simulink model "CL_NL_DH_18_jun_2026"  (R2025b)
settings: Solver=ode4  StartTime=0.0  StopTime=150  FixedStep=Ts  RelTol=1e-3
values from neighbouring files (symbols this model uses):
  att_alt = 0    [guiagem_NL.m]
  coef_Ana = 1    [guiagem_NL.m]
  coef_Sato = 0    [guiagem_NL.m]
  i = find([Plantas.Ve] == VT_missao & [Plantas.He] == 600, 1)    [guiagem_NL.m]
  phi_psi = 0    [guiagem_NL.m]
  surfaces = 24    [guiagem_NL.m]
  Variacao_Iner = 0    [guiagem_NL.m]
  VT_Throttle = 1    [guiagem_NL.m]
undefined symbols (not defined in the file or in its folder): Plantas, refAlt, refPhi, refPsi, reftheta
libraries: simulink_extras x14
settings Model: SimulationMode=accelerator  Creator=mirko  LastModifiedBy=mirko

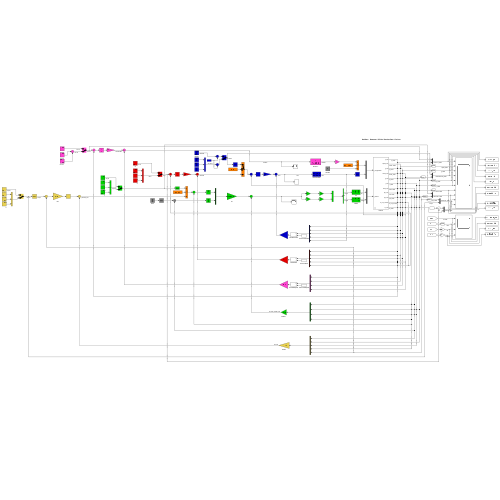
[thumbnail: Simulink's stored preview of the top-level diagram]
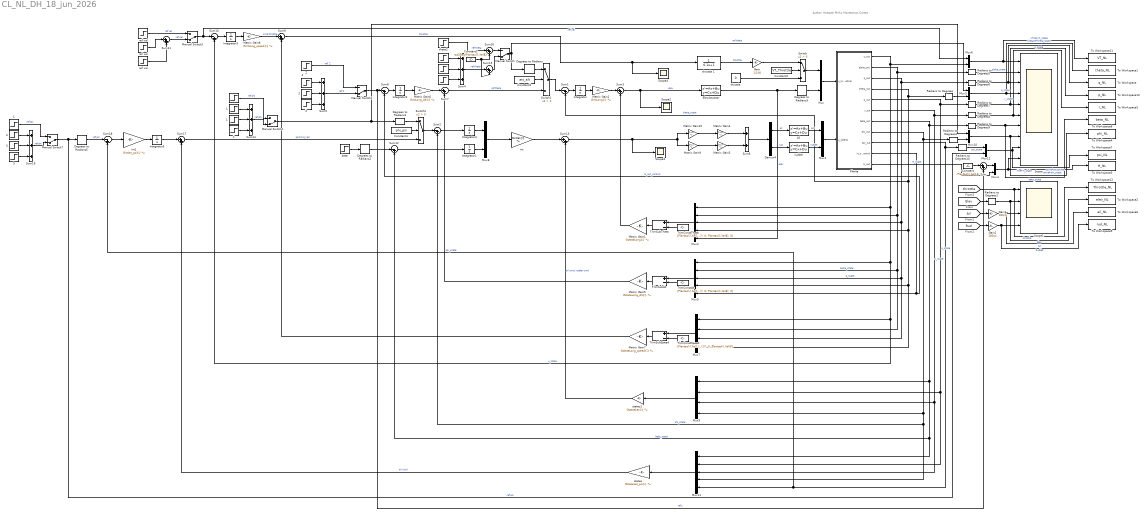
== system CL_NL_DH_18_jun_2026 ==
  note: Author: Huascar Mirko Montecinos Cortez
  "   " : Step  Time=80  After=refPhi  SampleTime=0
  "     " : Step  Time=40  After=reftheta  SampleTime=0
  "          " : Step  Time=80  Before=-reftheta  After=0  SampleTime=0
  "            " : Step  Time=60  Before=reftheta  After=-reftheta  SampleTime=0
  "            1" : Step  Time=110  Before=refPhi  After=-refPhi  SampleTime=0
  "            2" : Step  Time=60  Before=refAlt  After=-refAlt  SampleTime=0
  "            3" : Step  Time=110  Before=refPsi  After=-refPsi  SampleTime=0
  "          1" : Step  Time=130  Before=-refPhi  After=0  SampleTime=0
  "          2" : Step  Time=80  Before=-refAlt  After=0  SampleTime=0
  "          3" : Step  Time=130  Before=-refPsi  After=0  SampleTime=0
  "     1" : Step  Time=90  After=refPhi  SampleTime=0
  "     2" : Step  Time=40  After=refAlt  SampleTime=0
  "     3" : Step  Time=90  After=refPsi  SampleTime=0
  "   1" : Step  Time=80  After=refPsi  SampleTime=0
  " Z " : Step  Time=40  After=refAlt  SampleTime=0
  " ref vel " : Step  Time=5  Before=Plantas(i).Xe(1)  After=Plantas(i).Xe(1)  SampleTime=0
  Ail : StateSpace  A=-surfaces  B=surfaces  D=0  InitialCondition=0
  Constant : Constant  Value=-Plantas(i).Xe(12)
  Constant1 : Constant  Value=rad2deg(Plantas(i).Xe(8))
  Constant2 : Constant  Value=VT_Throttle
  Constant3 : Constant  Value=att_alt
  Constant4 : Constant  Value=phi_psi
  Degrees to Radians{,1..3,5} (5 alike) : simulink_extras/Transformations/Degrees to Radians
  Demux4 : Demux  Outputs=2
      settings: DisplayOption=none
  ElevActuator : StateSpace  A=-surfaces  B=surfaces  D=0  InitialCondition=Plantas(i).Ue(2)
  Gain : Gain  Gain=1/100
  Gain1 : Gain  Gain=180/pi
  Gain2 : Gain  Gain=180/pi
  Integrator{,1..5} (6 alike) : Integrator
  Manual Switch{,2..4,7} (5 alike) : ManualSwitch  CurrentSetting=0
  Matrix Gain1 : Gain  Gain=GstateLong{i}  Multiplication=Matrix(K*u)  SaturateOnIntegerOverflow=on  OutDataTypeStr=Inherit: Same as input  ParamDataTypeStr=Inherit: Same as input
  Matrix Gain10 : Gain  Gain=[1 0]  Multiplication=Matrix(K*u)  SaturateOnIntegerOverflow=on  OutDataTypeStr=Inherit: Same as input  ParamDataTypeStr=Inherit: Same as input
  Matrix Gain2 : Gain  Gain=GintLong{i}  Multiplication=Matrix(K*u)  SaturateOnIntegerOverflow=on  OutDataTypeStr=Inherit: Same as input  ParamDataTypeStr=Inherit: Same as input
  Matrix Gain3 : Gain  Gain=[0 1]'  Multiplication=Matrix(K*u)  SaturateOnIntegerOverflow=on  OutDataTypeStr=Inherit: Same as input  ParamDataTypeStr=Inherit: Same as input
  Matrix Gain4 : Gain  Gain=[1 0]'  Multiplication=Matrix(K*u)  SaturateOnIntegerOverflow=on  OutDataTypeStr=Inherit: Same as input  ParamDataTypeStr=Inherit: Same as input
  Matrix Gain5 : Gain  Gain=GstateLong_Alt{i}  Multiplication=Matrix(K*u)  SaturateOnIntegerOverflow=on  OutDataTypeStr=Inherit: Same as input  ParamDataTypeStr=Inherit: Same as input
  Matrix Gain6 : Gain  Gain=GintLong_Alt{i}  Multiplication=Matrix(K*u)  SaturateOnIntegerOverflow=on  OutDataTypeStr=Inherit: Same as input  ParamDataTypeStr=Inherit: Same as input
  Matrix Gain7 : Gain  Gain=GstateLong_speed{i}  Multiplication=Matrix(K*u)  SaturateOnIntegerOverflow=on  OutDataTypeStr=Inherit: Same as input  ParamDataTypeStr=Inherit: Same as input
  Matrix Gain8 : Gain  Gain=GintLong_speed{i}  Multiplication=Matrix(K*u)  SaturateOnIntegerOverflow=on  OutDataTypeStr=Inherit: Same as input  ParamDataTypeStr=Inherit: Same as input
  Matrix Gain9 : Gain  Gain=[0 1]  Multiplication=Matrix(K*u)  SaturateOnIntegerOverflow=on  OutDataTypeStr=Inherit: Same as input  ParamDataTypeStr=Inherit: Same as input
  Mux{,1,3..4,6,8,10,12} (8 alike) : Mux  Inputs=2
  Mux11 : Mux  Inputs=5
  Mux2 : Mux  Inputs=5
  Mux5 : Mux  Inputs=5
  Mux7 : Mux
  Mux9 : Mux
  Planta : Subsystem
  Radians to Degrees{,1,4..10} (9 alike) : simulink_extras/Transformations/Radians to Degrees
  Scope : Scope  NumInputPorts=10
      settings: ActiveDisplayString=10  ActiveDisplayYMinimum=593.67577098481627  ActiveDisplayYMaximum=606.307142927377
  Scope1 : Scope  NumInputPorts=4
      settings: ActiveDisplayString=4  ActiveDisplayYMinimum=-3.1238215479894382  ActiveDisplayYMaximum=4.435550961328742
  Scope2 : Scope
      settings: ActiveDisplayYMinimum=-1.3531942213324573  ActiveDisplayYMaximum=0.61662907005096645  DataLoggingVariableName=ScopeData2
  Scope3 : Scope
      settings: ActiveDisplayYMinimum=-0.008953837623387962  ActiveDisplayYMaximum=0.0080763644870395709  DataLoggingVariableName=ScopeData3
  Scope4 : Scope
      settings: ActiveDisplayYMinimum=-268.65761065429206  ActiveDisplayYMaximum=1519.894817061396  DataLoggingVariableName=ScopeData4
  Sum{,3,7,9,11,15..16} (7 alike) : Sum  Inputs=|++
  Sum1 : Sum  Inputs=|-+
  Sum10 : Sum  Inputs=|-+
  Sum12 : Sum  Inputs=|-+  SaturateOnIntegerOverflow=on
  Sum13 : Sum  Inputs=|++  SaturateOnIntegerOverflow=on
  Sum{4..5,14,19} (4 alike) : Sum  Inputs=+++
  Sum17 : Sum  Inputs=|++  SaturateOnIntegerOverflow=on
  Sum18 : Sum  Inputs=|-+  SaturateOnIntegerOverflow=on
  Sum2 : Sum  Inputs=|-+  SaturateOnIntegerOverflow=on
  Sum6 : Sum  Inputs=2  SaturateOnIntegerOverflow=on
  Sum8 : Sum  Inputs=|-+
  Switch : Switch  Criteria=u2 > Threshold  SaturateOnIntegerOverflow=off  InputSameDT=off
  Switch1 : Switch  Criteria=u2 > Threshold  SaturateOnIntegerOverflow=off  InputSameDT=off
  Switch2 : Switch  Criteria=u2 > Threshold  SaturateOnIntegerOverflow=off  InputSameDT=off
  To Workspace : ToWorkspace  VariableName=q_NL  SaveFormat=Structure With Time  SampleTime=-1
  To Workspace1 : ToWorkspace  VariableName=theta_NL  SaveFormat=Structure With Time  SampleTime=-1
  To Workspace10 : ToWorkspace  VariableName=p_NL  SaveFormat=Structure With Time  SampleTime=-1
  To Workspace11 : ToWorkspace  VariableName=VT_NL  SaveFormat=Structure With Time  SampleTime=-1
  To Workspace12 : ToWorkspace  VariableName=Throttle_NL  SaveFormat=Structure With Time  SampleTime=-1
  To Workspace2 : ToWorkspace  VariableName=elev_NL  SaveFormat=Structure With Time  SampleTime=-1
  To Workspace3 : ToWorkspace  VariableName=H_NL  SaveFormat=Structure With Time  SampleTime=-1
  To Workspace4 : ToWorkspace  VariableName=phi_NL  SaveFormat=Structure With Time  SampleTime=-1
  To Workspace5 : ToWorkspace  VariableName=r_NL  SaveFormat=Structure With Time  SampleTime=-1
  To Workspace6 : ToWorkspace  VariableName=ail_NL  SaveFormat=Structure With Time  SampleTime=-1
  To Workspace7 : ToWorkspace  VariableName=psi_NL  SaveFormat=Structure With Time  SampleTime=-1
  To Workspace8 : ToWorkspace  VariableName=beta_NL  SaveFormat=Structure With Time  SampleTime=-1
  To Workspace9 : ToWorkspace  VariableName=rud_NL  SaveFormat=Structure With Time  SampleTime=-1
  TrimConstAlt : Constant  Value=[Plantas(i).Xe(1); atan(Plantas(i).Xe(3)/Plantas(i).Xe(1)); 0; Plantas(i).Xe(8); 0]  VectorParams1D=off
  TrimConstSpeed : Constant  Value=[Plantas(i).Xe(1); atan(Plantas(i).Xe(3)/Plantas(i).Xe(1)); 0; Plantas(i).Xe(8)]  VectorParams1D=off
  TrimConstTheta : Constant  Value=[Plantas(i).Xe(1); atan(Plantas(i).Xe(3)/Plantas(i).Xe(1)); 0; Plantas(i).Xe(8); 0]  VectorParams1D=off
  TrimSubAlt : Sum  Inputs=+-
  TrimSubSpeed : Sum  Inputs=+-
  TrimSubTheta : Sum  Inputs=+-
  beta : Step  Time=0  After=0  SampleTime=0
  int : Gain  Gain=Gintlat{i}  Multiplication=Matrix(K*u)  SaturateOnIntegerOverflow=on  OutDataTypeStr=Inherit: Same as input  ParamDataTypeStr=Inherit: Same as input
  int1 : Gain  Gain=Gintlat_psi{i}  Multiplication=Matrix(K*u)  SaturateOnIntegerOverflow=on  OutDataTypeStr=Inherit: Same as input  ParamDataTypeStr=Inherit: Same as input
  ref vel : Step  Time=10  Before=Plantas(i).Xe(1)  After=Plantas(i).Xe(1)+3  SampleTime=0
  "ref vel  " : Step  Time=20  After=-3  SampleTime=0
  rudder : StateSpace  A=-surfaces  B=surfaces  D=0  InitialCondition=0
  states : Gain  Gain=GstateLat_psi{i}  Multiplication=Matrix(K*u)  SaturateOnIntegerOverflow=on  OutDataTypeStr=Inherit: Same as input  ParamDataTypeStr=Inherit: Same as input
  states1 : Gain  Gain=GstateLat{i}  Multiplication=Matrix(K*u)  SaturateOnIntegerOverflow=on  OutDataTypeStr=Inherit: Same as input  ParamDataTypeStr=Inherit: Same as input
  theta2 : Step  Time=100  After=reftheta  SampleTime=0
  throttle : Constant  Value=0
  throttle 1 : TransferFcn  Denominator=[0.1 1]
  wires:
  Mux/1 -> Planta/1(u_longitudinal)
  Mux1/1 -> Planta/2(u_lateral)
  Manual Switch/1 -> Degrees to Radians/1, Mux3/1  "ref theta"
  Matrix Gain1/1 -> Sum3/2
  Matrix Gain2/1 -> Sum3/1
  Integrator/1 -> Matrix Gain2/1
  Sum4/1 -> Sum15/1  "ref theta"
  Sum1/1 -> Integrator/1
  Switch1/1 -> Sum1/1
  theta2/1 -> Sum16/1  "ref theta"
  Sum3/1 -> Scope2/1, ElevActuator/1  "elev"
  Planta/1(u_out) -> Mux6/2, Mux7/1, Sum10/2, Mux5/1, Mux2/1  "u_state"
  Planta/2(alpha_out) -> Mux7/2, Mux5/2, Mux2/2, Radians to Degrees5/1  "alpha_state"
  Planta/3(q_out) -> Mux7/3, Mux5/3, Mux2/3, Radians to Degrees6/1  "q_state"
  Planta/4(theta_out) -> Mux7/4, Mux5/4, Mux2/4, Sum1/2, Radians to Degrees/1  "theta_state"
  Planta/5(p_out) -> Radians to Degrees7/1, Mux9/2, Mux11/2  "p_state"
  Planta/6(r_out) -> Radians to Degrees8/1, Mux9/3, Mux11/3  "r_state"
  Planta/7(beta_out) -> Radians to Degrees9/1, Mux11/1, Sum12/2, Mux9/1  "beta_state"
  Planta/8(phi_out) -> Radians to Degrees4/1, Mux11/4, Sum2/2, Mux9/4  "phi_state"
  Planta/9(psi_out) -> Mux11/5, Sum18/2, Radians to Degrees10/1  "psi_state"
  Planta/10(H_out_control) -> Mux5/5, Sum8/2  "H_out_control"
  Mux3/1 -> To Workspace1/1, Scope/4  "thetaref-theta_state"
  Radians to Degrees/1 -> Mux3/2
  Matrix Gain5/1 -> Sum7/2
  " Z "/1 -> Manual Switch2/1  "ref  Z"
  Manual Switch2/1 -> Sum8/1, Sum/2  "ref z"
  Sum8/1 -> Integrator2/1
  Sum7/1 -> Switch1/3  "ref theta"
  Sum5/1 -> Manual Switch2/2  "ref Z"
  Matrix Gain6/1 -> Sum7/1
  Integrator2/1 -> Matrix Gain6/1
  Degrees to Radians/1 -> Switch1/1
  Mux4/1 -> Scope/10, To Workspace3/1  "Href-H_state"
  Constant/1 -> Sum/1
  Sum/1 -> Mux4/1
  Radians to Degrees1/1 -> Scope1/2, To Workspace2/1  "Elev"
  Gain1/1 -> Scope1/3, To Workspace6/1  "Ail"
  Gain2/1 -> Scope1/4, To Workspace9/1  "Rudder"
  "ref vel  "/1 -> Sum11/2
  Sum10/1 -> Integrator3/1
  ref vel/1 -> Sum11/1
  Matrix Gain7/1 -> Sum9/2
  " ref vel "/1 -> Manual Switch3/1  "ref vel"
  Manual Switch3/1 -> Mux6/1, Sum10/1  "ref vel"
  Integrator3/1 -> Matrix Gain8/1
  Sum11/1 -> Manual Switch3/2  "ref vel"
  Matrix Gain8/1 -> Sum9/1  "cmd throttle"
  [Elev] -> Radians to Degrees1/1
  [Ail] -> Gain1/1
  [Rud] -> Gain2/1
  [throttle] -> To Workspace12/1, Scope1/1  "throttle"
  Sum9/1 -> Scope4/1, throttle 1/1  "throttle"
  Mux6/1 -> To Workspace11/1, Scope/1  "VTref-VT_state"
  Matrix Gain9/1 -> Matrix Gain3/1
  Matrix Gain10/1 -> Matrix Gain4/1
  Matrix Gain4/1 -> Sum6/1
  Sum13/1 -> Scope3/1, Matrix Gain9/1, Matrix Gain10/1
  Matrix Gain3/1 -> Sum6/2
  Sum6/1 -> Demux4/1
  Demux4/2 -> rudder/1  "rud"
  Demux4/1 -> Ail/1  "ail"
  beta/1 -> Degrees to Radians2/1
  "   "/1 -> Manual Switch4/1  "ref phi"
  int/1 -> Sum13/1
  Degrees to Radians2/1 -> Sum12/1
  Mux8/1 -> int/1
  Sum12/1 -> Integrator1/1
  "     1"/1 -> Sum14/1
  Sum14/1 -> Manual Switch4/2  "ref phi"
  "            1"/1 -> Sum14/2
  "          1"/1 -> Sum14/3
  Integrator4/1 -> Mux8/1
  Integrator1/1 -> Mux8/2
  Sum2/1 -> Integrator4/1
  Mux9/1 -> states1/1
  states1/1 -> Sum13/2  "ail cmd, rudder cmd"
  Mux10/1 -> To Workspace4/1, Scope/8  "phiref-phi_state"
  Radians to Degrees4/1 -> Mux10/2
  Manual Switch4/1 -> Mux10/1, Degrees to Radians1/1
  throttle/1 -> Switch/3
  Radians to Degrees5/1 -> Scope/2  "alpha_state"
  Radians to Degrees6/1 -> To Workspace/1, Scope/3  "q_state"
  Radians to Degrees7/1 -> To Workspace10/1, Scope/5  "p_state"
  Radians to Degrees8/1 -> Scope/6, To Workspace5/1  "r_state"
  Radians to Degrees9/1 -> Scope/7, To Workspace8/1  "beta_state"
  Degrees to Radians3/1 -> Mux/2
  Gain/1 -> Switch/1
  Mux12/1 -> To Workspace7/1, Scope/9  "psiref-psi_state"
  Planta/11(H_out) -> Mux4/2  "H_state"
  Constant1/1 -> Sum15/2, Sum16/2
  Sum15/1 -> Manual Switch/2
  Sum16/1 -> Manual Switch/1
  "          "/1 -> Sum4/3
  "     "/1 -> Sum4/1
  "            "/1 -> Sum4/2
  "          2"/1 -> Sum5/3
  "            2"/1 -> Sum5/2
  "     2"/1 -> Sum5/1
  Mux11/1 -> states/1
  Sum18/1 -> int1/1
  Integrator5/1 -> Sum17/1
  Manual Switch7/1 -> Degrees to Radians5/1, Mux12/2  "ref psi"
  int1/1 -> Integrator5/1
  Sum17/1 -> Switch2/3  "psiCmd_rad"
  states/1 -> Sum17/2  "ail cmd"
  Switch2/1 -> Sum2/1
  Degrees to Radians1/1 -> Switch2/1
  "     3"/1 -> Sum19/1
  "            3"/1 -> Sum19/2
  "   1"/1 -> Manual Switch7/1  "ref psi"
  Sum19/1 -> Manual Switch7/2  "ref phi"
  "          3"/1 -> Sum19/3
  Radians to Degrees10/1 -> Mux12/1  "psi_state"
  Degrees to Radians5/1 -> Sum18/1  "ref psi"
  Constant2/1 -> Switch/2
  Constant3/1 -> Switch1/2
  Constant4/1 -> Switch2/2
  Mux7/1 -> TrimSubSpeed/1
  TrimConstSpeed/1 -> TrimSubSpeed/2
  TrimSubSpeed/1 -> Matrix Gain7/1
  Mux2/1 -> TrimSubTheta/1
  TrimConstTheta/1 -> TrimSubTheta/2
  TrimSubTheta/1 -> Matrix Gain1/1
  Mux5/1 -> TrimSubAlt/1
  TrimConstAlt/1 -> TrimSubAlt/2
  TrimSubAlt/1 -> Matrix Gain5/1
  throttle 1/1 -> Gain/1  "throttle"
  rudder/1 -> Mux1/2  "rudder"
  Ail/1 -> Mux1/1  "Ail"
  ElevActuator/1 -> Degrees to Radians3/1, Mux2/5  "elev"
  Switch/1 -> Mux/1

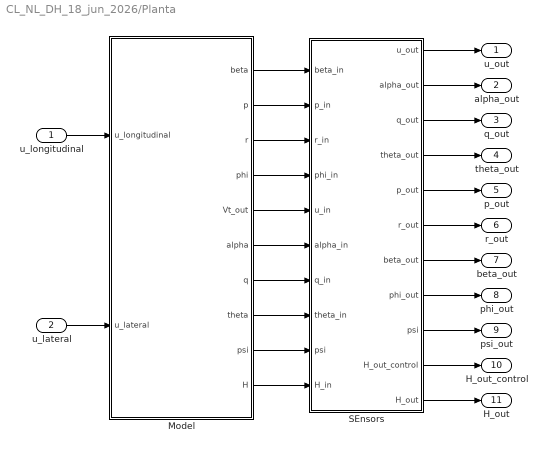
== system CL_NL_DH_18_jun_2026/Planta ==
  u_longitudinal : Inport
  u_lateral : Inport  Port=2
  Model : Subsystem
  SEnsors : Subsystem
  u_out : Outport
  alpha_out : Outport  Port=2
  q_out : Outport  Port=3
  theta_out : Outport  Port=4
  p_out : Outport  Port=5
  r_out : Outport  Port=6
  beta_out : Outport  Port=7
  phi_out : Outport  Port=8
  psi_out : Outport  Port=9
  H_out_control : Outport  Port=10
  H_out : Outport  Port=11
  wires:
  SEnsors/2(alpha_out) -> alpha_out/1
  SEnsors/3(q_out) -> q_out/1
  SEnsors/1(u_out) -> u_out/1
  Model/7(q) -> SEnsors/7(q_in)
  SEnsors/5(p_out) -> p_out/1
  Model/8(theta) -> SEnsors/8(theta_in)
  SEnsors/4(theta_out) -> theta_out/1
  u_lateral/1 -> Model/2(u_lateral)
  Model/1(beta) -> SEnsors/1(beta_in)
  SEnsors/6(r_out) -> r_out/1
  SEnsors/7(beta_out) -> beta_out/1
  Model/4(phi) -> SEnsors/4(phi_in)
  Model/5(Vt_out) -> SEnsors/5(u_in)
  SEnsors/9("psi ") -> psi_out/1
  Model/2(p) -> SEnsors/2(p_in)
  SEnsors/8(phi_out) -> phi_out/1
  Model/3(r) -> SEnsors/3(r_in)
  u_longitudinal/1 -> Model/1(u_longitudinal)
  Model/6(alpha) -> SEnsors/6(alpha_in)
  SEnsors/10(H_out_control) -> H_out_control/1
  Model/9(psi) -> SEnsors/9(psi)
  Model/10(H) -> SEnsors/10(H_in)
  SEnsors/11(H_out) -> H_out/1

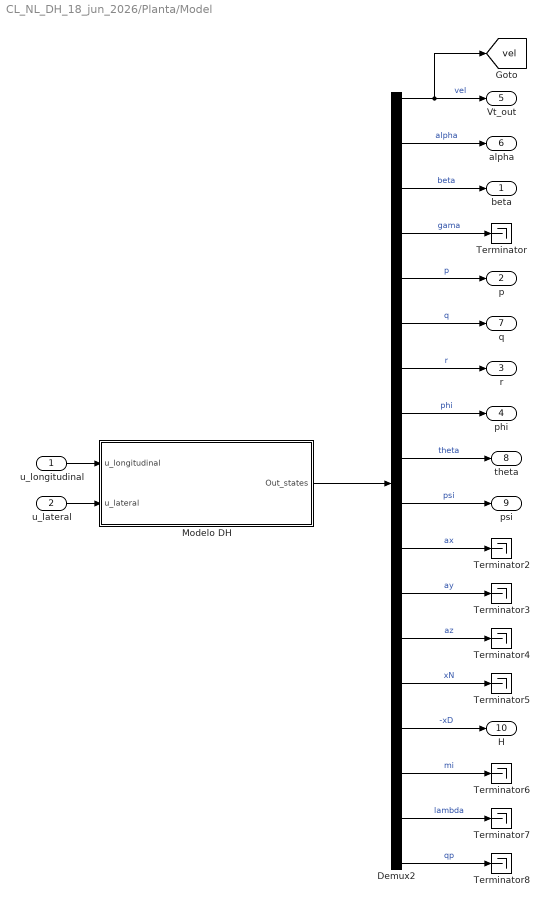
== system CL_NL_DH_18_jun_2026/Planta/Model ==
  u_longitudinal : Inport
  u_lateral : Inport  Port=2
  Demux2 : Demux  Outputs=18
  Modelo DH : Subsystem
  Terminator{,2..8} (8 alike) : Terminator
  beta : Outport
  p : Outport  Port=2
  r : Outport  Port=3
  phi : Outport  Port=4
  Vt_out : Outport  Port=5
  alpha : Outport  Port=6
  q : Outport  Port=7
  theta : Outport  Port=8
  psi : Outport  Port=9
  H : Outport  Port=10
  tag scope: vel=global
  wires:
  u_longitudinal/1 -> Modelo DH/1(u_longitudinal)
  Demux2/3 -> beta/1  "beta"
  Demux2/5 -> p/1  "p"
  Demux2/7 -> r/1  "r"
  Demux2/2 -> alpha/1  "alpha"
  Demux2/8 -> phi/1  "phi"
  Modelo DH/1(Out_states) -> Demux2/1
  Demux2/15 -> H/1  "-xD"
  Demux2/6 -> q/1  "q"
  u_lateral/1 -> Modelo DH/2(u_lateral)
  Demux2/4 -> Terminator/1  "gama"
  Demux2/10 -> psi/1  "psi"
  Demux2/11 -> Terminator2/1  "ax"
  Demux2/12 -> Terminator3/1  "ay"
  Demux2/13 -> Terminator4/1  "az"
  Demux2/14 -> Terminator5/1  "xN"
  Demux2/16 -> Terminator6/1  "mi"
  Demux2/17 -> Terminator7/1  "lambda"
  Demux2/18 -> Terminator8/1  "qp"
  Demux2/1 -> Vt_out/1, [vel]  "vel"
  Demux2/9 -> theta/1  "theta"

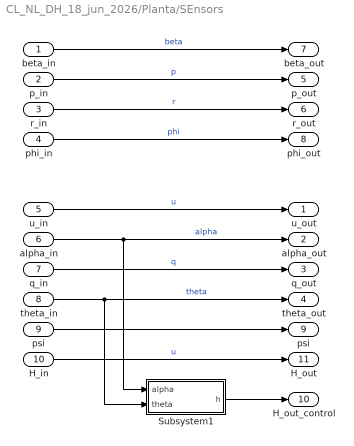
== system CL_NL_DH_18_jun_2026/Planta/SEnsors ==
  beta_in : Inport
  p_in : Inport  Port=2
  r_in : Inport  Port=3
  phi_in : Inport  Port=4
  u_in : Inport  Port=5
  alpha_in : Inport  Port=6
  q_in : Inport  Port=7
  theta_in : Inport  Port=8
  psi : Inport  Port=9
  H_in : Inport  Port=10
  Subsystem1 : Subsystem
  u_out : Outport
  alpha_out : Outport  Port=2
  q_out : Outport  Port=3
  theta_out : Outport  Port=4
  p_out : Outport  Port=5
  r_out : Outport  Port=6
  beta_out : Outport  Port=7
  phi_out : Outport  Port=8
  "psi " : Outport  Port=9
  H_out_control : Outport  Port=10
  H_out : Outport  Port=11
  wires:
  p_in/1 -> p_out/1  "p"
  phi_in/1 -> phi_out/1  "phi"
  r_in/1 -> r_out/1  "r"
  alpha_in/1 -> alpha_out/1, Subsystem1/1(alpha)  "alpha"
  beta_in/1 -> beta_out/1  "beta"
  u_in/1 -> u_out/1  "u"
  q_in/1 -> q_out/1  "q"
  theta_in/1 -> theta_out/1, Subsystem1/2(theta)  "theta"
  psi/1 -> "psi "/1
  Subsystem1/1(h) -> H_out_control/1
  H_in/1 -> H_out/1  "u"

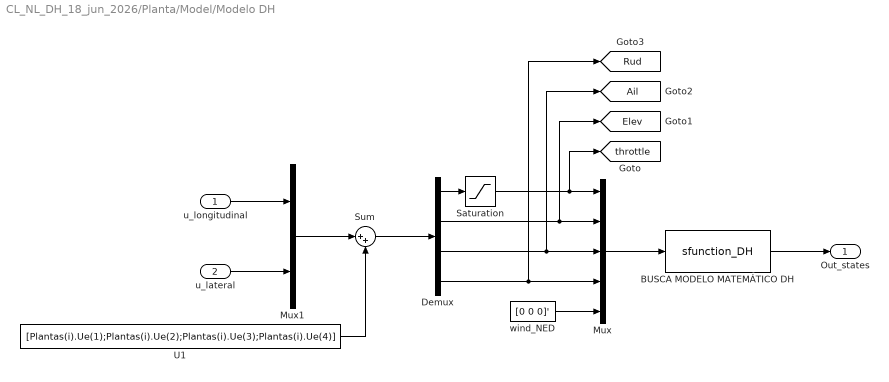
== system CL_NL_DH_18_jun_2026/Planta/Model/Modelo DH ==
  u_longitudinal : Inport
  u_lateral : Inport  Port=2
  "BUSCA MODELO MATEMÁTICO DH " : S-Function  FunctionName=sfunction_DH  Parameters=Plantas(i).Xe, coef_Sato, coef_Ana, Variacao_Iner  SFunctionDeploymentMode=off  EnableBusSupport=off
  Demux : Demux
  Mux : Mux  Inputs=5
  Mux1 : Mux  Inputs=2
  Saturation : Saturate  UpperLimit=1  LowerLimit=0
  Sum : Sum  Inputs=|++
  U1 : Constant  Value=[Plantas(i).Ue(1);Plantas(i).Ue(2);Plantas(i).Ue(3);Plantas(i).Ue(4)]
  wind_NED : Constant  Value=[0 0 0]'
  Out_states : Outport
  tag scope: Ail=global, Elev=global, Rud=global, throttle=global
  wires:
  "BUSCA MODELO MATEMÁTICO DH "/1 -> Out_states/1
  Mux1/1 -> Sum/1
  Sum/1 -> Demux/1
  u_lateral/1 -> Mux1/2
  u_longitudinal/1 -> Mux1/1
  wind_NED/1 -> Mux/5
  U1/1 -> Sum/2
  Demux/2 -> [Elev], Mux/2
  Demux/1 -> Saturation/1
  Demux/3 -> [Ail], Mux/3
  Demux/4 -> [Rud], Mux/4
  Mux/1 -> "BUSCA MODELO MATEMÁTICO DH "/1
  Saturation/1 -> [throttle], Mux/1

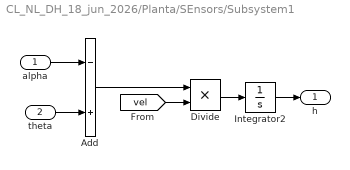
== system CL_NL_DH_18_jun_2026/Planta/SEnsors/Subsystem1 ==
  alpha : Inport
  theta : Inport  Port=2
  Add : Sum  Inputs=-+
  Divide : Product  Inputs=**
  Integrator2 : Integrator
  h : Outport
  wires:
  Add/1 -> Divide/1
  Integrator2/1 -> h/1
  Divide/1 -> Integrator2/1
  alpha/1 -> Add/1
  theta/1 -> Add/2
  [vel] -> Divide/2
